simulink model "aaaqi"  (R2016b)
settings: Solver=ode4  StartTime=0.0  StopTime=inf  FixedStep=0.002  RelTol=1e-3  EnableMultiTasking=on
undefined symbols (not defined in the file or in its folder): bit, mdaadlink6208, sigbuilder_block, Standard
libraries: slrtlib x20, slrtsoftinglib x11, simulink x10
(part 4 of 4)

== stateflow chart aaaqi/Subsystem2/shoudong/Chart ==
  state shoudong
    state kaiguangai [parallel]
      settings: executionOrder=1
      state start
        entry:
        xuansong=0;
        xuanjin=0;
        suoding=0;
        jiesuo=0;
        kaigaikaishi=0;
        guangaikaishi=0;
        diancifa20=0;
      state on1
        entry:diancifa20=1;
      state on5
        entry:
        jiesuo=1;
      state on2
        entry:
        xuansong=1;
      state off10
        entry:
        jiesuo=0;
      state off8
        entry:
        xuansong=0;
      state off5
        entry:
        jiesuo=0;
      state off1
        entry:
        xuansong=0;
      state on6
        entry:
        guangaikaishi=1;
      state off2
        entry:
        diancifa20=0;
        SQshiyabuchangwancheng=1;
      state on73
        entry:
        guangaikaishi=0;
      state on7
        entry:
        guangaikaishi=0;
      state on3
        entry:
        kaigaikaishi=1;
      state on71
        entry:
        diancifa20=1;
      state on72
        entry:
        kaigaikaishi=0;
      state on8
        entry:
        xuanjin=1;
      state on4
        entry:
        kaigaikaishi=0;
      state off11
        entry:
        xuanjin=0;
      state on41
        entry:
        suoding=1;
      state off6
        entry:
        xuanjin=0;
      state off9
        entry:
        suoding=0;
      state off3
        entry:
        suoding=0;
      state off7
        entry:
        diancifa20=0;
        SQxuanjinjianyawancheng=1;
        guangaiwancheng=1;
      state off4
        entry:
        kaigaiwancheng=1;
      (default) -> shoudong.kaiguangai.start
      off7 -> shoudong.kaiguangai.start
      shoudong.kaiguangai.start -> shoudong.kaiguangai.on1 : [shiyabuchang==1]
      shoudong.kaiguangai.off4 -> shoudong.kaiguangai.on5 : [jiesuomingling==1]
      off10 -> shoudong.kaiguangai.on5 : [jiesuomingling==1]
      shoudong.kaiguangai.on5 -> (junction 1244)
      shoudong.kaiguangai.on1 -> shoudong.kaiguangai.on2 : [liuliangji==1&&p1>=p2-0.01&&p1<=p2+0.01&&xuansongmingling==1]
      off8 -> shoudong.kaiguangai.on2 : [xuansongmingling==1]
      (junction 1244) -> off10 [order 2] : [jiesuomingling==0]
      (junction 1244) -> off5 [order 1] : [jiesuodaowei1==1&&jiesuodaowei2==1]
      shoudong.kaiguangai.on2 -> (junction 1245)
      (junction 1245) -> off8 [order 2] : [xuansongmingling==0]
      (junction 1245) -> shoudong.kaiguangai.off1 [order 1] : [xuansongdaowei1==1&&xuansongdaowei2==1]
      off5 -> shoudong.kaiguangai.on6 : after(500,tick)[guangai==1]
      shoudong.kaiguangai.off1 -> shoudong.kaiguangai.off2 : after(200,tick)
      on73 -> shoudong.kaiguangai.on6 : [guangai==1]
      shoudong.kaiguangai.on6 -> (junction 1246)
      (junction 1246) -> on73 [order 2] : [guangai==0]
      (junction 1246) -> on7 [order 1] : [guangaijieshu==1]
      shoudong.kaiguangai.off2 -> shoudong.kaiguangai.on3 : after(500,tick)[kaigai==1]
      on7 -> on71 : [xuanjinjianya==1]
      on72 -> shoudong.kaiguangai.on3 : [kaigai==1]
      shoudong.kaiguangai.on3 -> (junction 1247)
      on71 -> on8 : [xuanjinmingling==1]
      (junction 1247) -> on72 [order 2] : [kaigai==0]
      (junction 1247) -> shoudong.kaiguangai.on4 [order 1] : [kaigaijieshu==1]
      off11 -> on8 : [xuanjinmingling==1]
      on8 -> (junction 1248)
      shoudong.kaiguangai.on4 -> on41 : [suodingmingling==1]
      (junction 1248) -> off11 [order 2] : [xuanjinmingling==0]
      (junction 1248) -> shoudong.kaiguangai.off6 [order 1] : [xuanjindaowei1==1&&xuanjindaowei2==1]
      off9 -> on41 : [suoding==1]
      on41 -> (junction 1249)
      (junction 1249) -> off9 [order 2] : [suoding==0]
      (junction 1249) -> shoudong.kaiguangai.off3 [order 1] : [suodingdaowei1==1&&suodingdaowei2==1]
      shoudong.kaiguangai.off6 -> off7 : after(200,tick)
      shoudong.kaiguangai.off3 -> shoudong.kaiguangai.off4 : after(200,tick)
    state SXQxieya [parallel]
      settings: executionOrder=4
      state off1
        entry:
        diancifa11_1=0;
        diancifa11_5=0;
        bililiuliangfa18_1=0;
        bililiuliangfa18_2=0;
        bililiuliangfa18_3=0;
        bililiuliangfa18_4=0;
      state on1
        entry:
        diancifa11_5=1;
      state xieya1
        entry:
        bililiuliangfa18_1=1;
        bililiuliangfa18_2=1;
        p0_2=p0sheding;
      state xieya1_1
        entry:
        bililiuliangfa18_1=1;
        bililiuliangfa18_2=1;
      state xieya1_2
        entry:
        bililiuliangfa18_1=1;
        bililiuliangfa18_2=0;
      state xieya2
        entry:
        bililiuliangfa18_1=1;
        bililiuliangfa18_2=1;
        p0_2=p0_2-0.03;
      state xieya1_3
        entry:
        bililiuliangfa18_1=0;
        bililiuliangfa18_2=1;
      state xieya7_1
        entry:
        bililiuliangfa18_1=1;
        bililiuliangfa18_2=1;
      state xieya7_2
        entry:
        bililiuliangfa18_1=1;
        bililiuliangfa18_2=0;
      state xieya8
        entry:
        bililiuliangfa18_1=1;
        bililiuliangfa18_2=1;
      state xieya7_3
        entry:
        bililiuliangfa18_1=0;
        bililiuliangfa18_2=1;
      state off2
        entry:
        diancifa11_5=0;
        bililiuliangfa18_1=0;
        bililiuliangfa18_2=0;
        SXQxieyawancheng=1;
      (default) -> shoudong.SXQxieya.off1
      (junction 1418) -> shoudong.SXQxieya.off1
      (junction 1419) -> shoudong.SXQxieya.off1
      (junction 1421) -> (junction 1418) [order 2] : [SXQxieya==0]
      (junction 1424) -> (junction 1418) [order 2] : [SXQxieya==0]
      (junction 1420) -> (junction 1418) [order 2] : [SXQxieya==0]
      (junction 1423) -> (junction 1418) [order 2] : [SXQxieya==0]
      (junction 1426) -> (junction 1419) [order 2] : [SXQxieya==0]
      (junction 1429) -> (junction 1419) [order 2] : [SXQxieya==0]
      (junction 1427) -> (junction 1419) [order 2] : [SXQxieya==0]
      (junction 1430) -> (junction 1419) [order 2] : [SXQxieya==0]
      shoudong.SXQxieya.off1 -> shoudong.SXQxieya.on1 : [SXQxieya==1]
      shoudong.SXQxieya.on1 -> xieya1 : after(500,tick)
      xieya1 -> (junction 1422)
      (junction 1422) -> (junction 1421) [order 2] : [p2<=p0_2&&p3>p0_2]
      (junction 1420) -> xieya1_1 [order 1] : [SXQxieya==1]
      (junction 1421) -> xieya1_2 [order 1] : [SXQxieya==1]
      (junction 1422) -> (junction 1420) [order 1] : [p2>p0_2&&p3>p0_2]
      xieya1_2 -> (junction 1422)
      xieya1_1 -> (junction 1422)
      xieya1_3 -> (junction 1422)
      (junction 1422) -> (junction 1423) [order 4] : [p2<=p0_2&&p3<=p0_2]
      (junction 1422) -> (junction 1424) [order 3] : [p2>p0_2&&p3<=p0_2]
      (junction 1425) -> (junction 1422) [order 2] : [p0_2>p0_0]
      (junction 1423) -> xieya2 [order 1] : [SXQxieya==1]
      (junction 1424) -> xieya1_3 [order 1] : [SXQxieya==1]
      xieya2 -> (junction 1425)
      (junction 1425) -> (junction 1428) [order 1] : [p0_2<=p0_0]
      (junction 1427) -> xieya7_2 [order 1] : [SXQxieya==1]
      (junction 1426) -> xieya7_1 [order 1] : [SXQxieya==1]
      (junction 1428) -> (junction 1427) [order 2] : [p2<=p0_0&&p3>p0_0]
      (junction 1428) -> (junction 1426) [order 1] : [p2>p0_0&&p3>p0_0]
      xieya7_1 -> (junction 1428)
      xieya7_2 -> (junction 1428)
      (junction 1428) -> (junction 1430) [order 3] : [p2>p0_0&&p3<=p0_0]
      (junction 1428) -> (junction 1429) [order 4] : [p2<=p0_0&&p3<=p0_0]
      xieya7_3 -> (junction 1428)
      (junction 1431) -> (junction 1428) [order 2] : [p2>p0_0||p3>p0_0]
      (junction 1429) -> xieya8 [order 1] : [SXQxieya==1]
      (junction 1430) -> xieya7_3 [order 1] : [SXQxieya==1]
      xieya8 -> (junction 1431) : after(1000,tick)
      (junction 1431) -> shoudong.SXQxieya.off2 [order 1] : [p2<=p0_0&&p3<=p0_0]
    state SCjiaya [parallel]
      settings: executionOrder=2
      state off1
        entry:diancifa11_1=0;
        diancifa11_2=0;
        diancifa16_1=0;
      state on1
        entry:diancifa11_1=1;
        diancifa11_2=1;
        diancifa16_1=0;
      state off2
        entry:
        diancifa11_1=0;
        diancifa11_2=0;
        diancifa16_1=0;
      state on3
        entry:diancifa11_1=1;
        diancifa11_2=1;
        diancifa16_1=0;
      state on2
        entry:diancifa16_1=1;
      state off3
        entry:
        diancifa11_1=0;
        diancifa11_2=0;
        diancifa16_1=0;
      state off4
        entry:
        SCjiayawancheng=1;
      (default) -> shoudong.SCjiaya.off1
      (junction 1311) -> shoudong.SCjiaya.off1
      shoudong.SCjiaya.off1 -> shoudong.SCjiaya.on1 : [SCjiaya==1]
      shoudong.SCjiaya.on1 -> (junction 1312)
      (junction 1312) -> (junction 1311) [order 2] : [SCjiaya==0]
      (junction 1313) -> (junction 1311) [order 2] : [SCjiaya==0]
      (junction 1312) -> shoudong.SCjiaya.off2 [order 1] : [p1>=p1sheding]
      shoudong.SCjiaya.off2 -> (junction 1313)
      shoudong.SCjiaya.on3 -> (junction 1314)
      (junction 1313) -> (junction 1314) [order 1] : after(1000,tick)
      shoudong.SCjiaya.on2 -> (junction 1314)
      (junction 1314) -> shoudong.SCjiaya.on2 [order 2] : [p1>p1sheding+0.005]
      (junction 1314) -> shoudong.SCjiaya.on3 [order 1] : [p1<p1sheding]
      (junction 1314) -> shoudong.SCjiaya.off3 [order 3] : [p1>=p1sheding&&p1<=p1sheding+0.005]
      shoudong.SCjiaya.off3 -> shoudong.SCjiaya.off4
    state SCzhushui [parallel]
      settings: executionOrder=3
      state off4
        entry:diancifa16_1=0;
        diancifa3=0;
      state on2
        entry:diancifa16_1=1;
      state on3
        entry:diancifa3=1;
      state off1
        entry:diancifa3=0;
      state off2
        entry:diancifa16_1=0;
      state off3
        entry:
        SCzhushuiwancheng=1;
      (default) -> shoudong.SCzhushui.off4
      (junction 1338) -> shoudong.SCzhushui.off4 [order 2] : [SCzhushui==0]
      shoudong.SCzhushui.off4 -> shoudong.SCzhushui.on2 : [SCzhushui==1]
      shoudong.SCzhushui.on2 -> shoudong.SCzhushui.on3 : after(20,tick)
      shoudong.SCzhushui.on3 -> (junction 1338)
      (junction 1338) -> shoudong.SCzhushui.off1 [order 1] : [fuqiuyeweikongzhiqi==1]
      shoudong.SCzhushui.off1 -> shoudong.SCzhushui.off2
      shoudong.SCzhushui.off2 -> shoudong.SCzhushui.off3
    state SXQjunya [parallel]
      settings: executionOrder=5
      state jiaya1_1
        entry:
        bililiuliangfa18_3=1;
        bililiuliangfa18_4=1;
      state jiaya7_1
        entry:
        bililiuliangfa18_3=1;
        bililiuliangfa18_4=1;
      state jiaya7_3
        entry:
        bililiuliangfa18_3=0;
        bililiuliangfa18_4=1;
      state on6
        entry:
        bililiuliangfa18_3=1;
        diancifa3=1;
        p0_1=p0_1+0.02;
      state on5
        entry:
        bililiuliangfa18_3=1;
        diancifa3=1;
      state jiaya2
        entry:
        bililiuliangfa18_3=1;
        bililiuliangfa18_4=1;
        p0_1=p0_1+0.03;
      state off1
        entry:
        diancifa11_1=0;
        diancifa11_5=0;
        diancifa20=0;
        diancifa3=0;
        bililiuliangfa18_1=0;
        bililiuliangfa18_2=0;
        bililiuliangfa18_3=0;
        bililiuliangfa18_4=0;
      state jiaya1
        entry:
        diancifa3=0;
        bililiuliangfa18_3=1;
        bililiuliangfa18_4=1;
        p0_1=p0sheding_qi;
      state on1
        entry:
        diancifa11_1=1;
      state on2
        entry:
        bililiuliangfa18_3=1;
        diancifa3=1;
      state jiaya7_2
        entry:
        bililiuliangfa18_3=1;
        bililiuliangfa18_4=0;
      state jiaya1_2
        entry:
        bililiuliangfa18_3=1;
        bililiuliangfa18_4=0;
      state on3
        entry:
        bililiuliangfa18_3=0;
        diancifa3=1;
      state on4
        entry:
        bililiuliangfa18_3=1;
        diancifa3=0;
      state jiaya1_3
        entry:
        bililiuliangfa18_3=0;
        bililiuliangfa18_4=1;
      state off4
        entry:
        bililiuliangfa18_3=0;
        bililiuliangfa18_4=0;
      state off3
        entry:
        bililiuliangfa18_1=0;
        bililiuliangfa18_2=0;
      state off2
        entry:
        bililiuliangfa18_1=0;
        bililiuliangfa18_2=0;
        bililiuliangfa18_3=0;
        bililiuliangfa18_4=0;
      state jiance1_34
        entry:
        bililiuliangfa18_1=1;
        bililiuliangfa18_2=0;
      state jiance1_32
        entry:
        bililiuliangfa18_1=1;
        bililiuliangfa18_2=1;
      state jiance1_36
        entry:
        bililiuliangfa18_1=0;
        bililiuliangfa18_2=1;
      state off6
        entry:
        diancifa11_1=0;
        diancifa11_5=0;
        SXQjunyawancheng=1;
      jiaya1_1 -> (junction 1492)
      (junction 1683) -> shoudong.SXQjunya.on6 [order 1] : [SXQjunya==1]
      jiaya7_3 -> (junction 1494)
      shoudong.SXQjunya.on5 -> (junction 1665)
      (junction 1488) -> jiaya2 [order 1] : [SXQjunya==1]
      (junction 1487) -> jiaya7_1 [order 1] : [SXQjunya==1]
      (default) -> shoudong.SXQjunya.off1
      (junction 1490) -> jiaya1_1 [order 1] : [SXQjunya==1]
      jiaya7_1 -> (junction 1494)
      (junction 1489) -> jiaya7_3 [order 1] : [SXQjunya==1]
      (junction 1684) -> shoudong.SXQjunya.on5 [order 1] : [SXQjunya==1]
      shoudong.SXQjunya.on6 -> (junction 1676)
      (junction 1487) -> (junction 1499) [order 2] : [SXQjunya==0]
      (junction 1494) -> (junction 1487) [order 1] : [p2<p0sheding&&p3<p0sheding]
      jiaya2 -> (junction 1493)
      (junction 1665) -> (junction 1683) [order 4] : [p2>=p0_1&&p3>=p0_1]
      (junction 1683) -> (junction 1666) [order 2] : [SXQjunya==0]
      (junction 1492) -> (junction 1488) [order 4] : [p2>=p0_1&&p3>=p0_1]
      (junction 1488) -> (junction 1498) [order 2] : [SXQjunya==0]
      (junction 1489) -> (junction 1499) [order 2] : [SXQjunya==0]
      (junction 1494) -> (junction 1489) [order 3] : [p2<p0sheding&&p3>=p0sheding]
      (junction 1665) -> (junction 1684) [order 1] : [p2<p0_1&&p3<p0_1]
      (junction 1492) -> (junction 1490) [order 1] : [p2<p0_1&&p3<p0_1]
      (junction 1490) -> (junction 1498) [order 2] : [SXQjunya==0]
      (junction 1684) -> (junction 1666) [order 2] : [SXQjunya==0]
      (junction 1494) -> (junction 1491) [order 2] : [p2>=p0sheding&&p3<p0sheding]
      (junction 1491) -> (junction 1499) [order 2] : [SXQjunya==0]
      (junction 1491) -> jiaya7_2 [order 1] : [SXQjunya==1]
      jiaya1 -> (junction 1492)
      (junction 1493) -> (junction 1492) [order 2] : [p0_1<p0sheding]
      (junction 1493) -> (junction 1494) [order 1] : [p0_1>=p0sheding]
      shoudong.SXQjunya.on1 -> shoudong.SXQjunya.on2 : after(500,tick)
      (junction 1492) -> (junction 1496) [order 3] : [p2<p0_1&&p3>=p0_1]
      jiaya7_2 -> (junction 1494)
      jiaya1_3 -> (junction 1492)
      shoudong.SXQjunya.on2 -> (junction 1665)
      (junction 1676) -> (junction 1665) [order 2] : [p0_1<=p0sheding_qi]
      (junction 1676) -> jiaya1 [order 1] : [p0_1>p0sheding_qi]
      shoudong.SXQjunya.off3 -> (junction 1494) [order 2] : [p2<=(p0sheding+0.005)&&p3<=(p0sheding+0.005)]
      (junction 1492) -> (junction 1495) [order 2] : [p2>=p0_1&&p3<p0_1]
      shoudong.SXQjunya.off1 -> shoudong.SXQjunya.on1 : [SXQjunya==1]
      shoudong.SXQjunya.off4 -> (junction 1494) [order 2] : [p2<p0sheding||p3<p0sheding]
      jiaya1_2 -> (junction 1492)
      (junction 1494) -> (junction 1497) [order 4] : after(250,tick)[p2>=p0sheding&&p3>=p0sheding]
      (junction 1665) -> (junction 1670) [order 2] : [p2<p0_1&&p3>=p0_1]
      (junction 1665) -> (junction 1680) [order 3] : [p2>=p0_1&&p3<p0_1]
      shoudong.SXQjunya.on4 -> (junction 1665)
      shoudong.SXQjunya.on3 -> (junction 1665)
      (junction 1495) -> jiaya1_2 [order 1] : [SXQjunya==1]
      (junction 1495) -> (junction 1498) [order 2] : [SXQjunya==0]
      (junction 1496) -> jiaya1_3 [order 1] : [SXQjunya==1]
      (junction 1680) -> shoudong.SXQjunya.on4 [order 1] : [SXQjunya==1]
      (junction 1496) -> (junction 1498) [order 2] : [SXQjunya==0]
      (junction 1680) -> (junction 1666) [order 2] : [SXQjunya==0]
      (junction 1670) -> shoudong.SXQjunya.on3 [order 1] : [SXQjunya==1]
      (junction 1670) -> (junction 1666) [order 2] : [SXQjunya==0]
      (junction 1666) -> shoudong.SXQjunya.off1
      (junction 1497) -> (junction 1499) [order 2] : [SXQjunya==0]
      (junction 1497) -> shoudong.SXQjunya.off4 [order 1] : [SXQjunya==1]
      (junction 1500) -> shoudong.SXQjunya.off3 [order 1] : [SXQjunya==1]
      (junction 1499) -> (junction 1498)
      (junction 1498) -> (junction 1666)
      (junction 1501) -> (junction 1499)
      shoudong.SXQjunya.off3 -> (junction 1503) [order 1] : [p2>(p0sheding+0.005)||p3>(p0sheding+0.005)]
      shoudong.SXQjunya.off4 -> (junction 1503) [order 1]
      (junction 1500) -> (junction 1501) [order 2] : [SXQjunya==0]
      (junction 1503) -> (junction 1500) [order 5] : after(250,tick)[p2<=(p0sheding+0.005)&&p3<=(p0sheding+0.005)]
      (junction 1502) -> (junction 1501) [order 2] : [SXQjunya==0]
      (junction 1504) -> (junction 1501) [order 2] : [SXQjunya==0]
      (junction 1506) -> (junction 1501) [order 2] : [SXQjunya==0]
      (junction 1503) -> (junction 1502) [order 1] : [p2<=(p0sheding+0.005)&&p3>(p0sheding+0.005)]
      (junction 1502) -> jiance1_34 [order 1] : [SXQjunya==1]
      (junction 1503) -> shoudong.SXQjunya.off2 [order 2] : [p2>=p0sheding&&p3>=p0sheding&&p2<=(p0sheding+0.005)&&p3<=(p0sheding+0.005)]
      jiance1_34 -> (junction 1503)
      (junction 1505) -> (junction 1503) [order 1] : [p2<p0sheding||p2>(p0sheding+0.005)||p3<p0sheding||p3>(p0sheding+0.005)]
      jiance1_32 -> (junction 1503)
      (junction 1503) -> (junction 1504) [order 3] : [p2>(p0sheding+0.005)&&p3<=(p0sheding+0.005)]
      jiance1_36 -> (junction 1503)
      (junction 1503) -> (junction 1506) [order 4] : [p2>(p0sheding+0.005)&&p3>(p0sheding+0.005)]
      shoudong.SXQjunya.off2 -> (junction 1505) : after(1000,tick)
      (junction 1504) -> jiance1_36 [order 1] : [SXQjunya==1]
      (junction 1505) -> shoudong.SXQjunya.off6 [order 2] : [p2>=p0sheding&&p2<=(p0sheding+0.005)&&p3>=p0sheding&&p3<=(p0sheding+0.005)]
      (junction 1506) -> jiance1_32 [order 1] : [SXQjunya==1]
  state start
    en:
    diancifa11_1=0;
    diancifa11_2=0;
    diancifa11_5=0;
    diancifa20=0;
    diancifa16_1=0;
    diancifa3=0;
    diancifa21=0;
    bililiuliangfa18_1=0;
    bililiuliangfa18_2=0;
    bililiuliangfa18_3=0;
    bililiuliangfa18_4=0;
    xuansong=0;
    xuanjin=0;
    suoding=0;
    jiesuo=0;
    kaigaikaishi=0;
    guangaikaishi=0;
  state off111
    en:
    diancifa11_1=0;
    diancifa11_2=0;
    diancifa11_5=0;
    diancifa20=0
    diancifa16_1=0;
    diancifa3=0;
    diancifa21=0;
    bililiuliangfa18_1=0;
    bililiuliangfa18_2=0;
    bililiuliangfa18_3=0;
    bililiuliangfa18_4=0;
    xuansong=0;
    xuanjin=0;
    suoding=0;
    jiesuo=0;
    SCzhushuiwancheng=0;
    SCjiayawancheng=0;
    SXQjunyawancheng=0;
    SQshiyabuchangwancheng=0;
    kaigaikaishi=0;
    kaigaiwancheng=0;
    SQxuanjinjianyawancheng=0;
    guangaikaishi=0;
    guangaiwancheng=0;
    SXQxieyawancheng=0;
  (default) -> start
  start -> shoudong : [start==1]
  off111 -> start : [start==0&&jiting==0]
  shoudong -> off111 : [jiting==1||start==0]
  data: start input double; diancifa11_1 output double; diancifa11_2 output double; diancifa11_5 output double; SCzhushui input double; fuqiuyeweikongzhiqi input double; diancifa20 output double; diancifa16_1 output double; diancifa3 output double; SCjiaya input double; SXQjunya input double; diancifa21 output double; suoding output double; jiesuo output double; xuansong output double; xuanjin output double; bililiuliangfa18_1 output double; bililiuliangfa18_2 output double; bililiuliangfa18_3 output double; bililiuliangfa18_4 output double; SXQxieya input double; p1 input double; p1sheding input double; liuliangji input double; p2 input double; p3 input double; p0_0 input double; p0sheding input double; kaigaikaishi output double; guangaikaishi output double; SCzhushuiwancheng output double; SCjiayawancheng output double; SXQjunyawancheng output double; SXQxieyawancheng output double; SQshiyabuchangwancheng output double; SQxuanjinjianyawancheng output double; kaigaiwancheng output double; guangaiwancheng output double; xuansongdaowei1 input double; xuansongdaowei2 input double; xuanjindaowei1 input double; xuanjindaowei2 input double; suodingdaowei1 input double; suodingdaowei2 input double; jiesuodaowei1 input double; jiesuodaowei2 input double; kaigaijieshu input double; guangaijieshu input double; jiting input double; kaigai input double; guangai input double; shiyabuchang input double; xuansongmingling input double; suodingmingling input double; jiesuomingling input double; xuanjinjianya input double; xuanjinmingling input double; p0_1 output double; p0_2 output double; p0sheding_qi input double

== stateflow chart aaaqi/guangaiquxian/Chart1 ==
  state on1
    en:
    x=0;
    t=0;
  state on2
    entry:
    x++;
    t=x*0.002
  (default) -> on1
  (junction 14) -> on1 [order 2] : [a==0]
  on1 -> on2 : [a==1]
  on2 -> (junction 14)
  (junction 14) -> on2 [order 1] : [a==1]
  data: a input double; x local double; t output double

== stateflow chart aaaqi/kaigaiquxian/Chart ==
  state on1
    en:
    x=0;
    t=0;
  state on2
    entry:
    x++;
    t=x*0.002
  (default) -> on1
  (junction 14) -> on1 [order 2] : [a==0]
  on1 -> on2 : [a==1]
  on2 -> (junction 14)
  (junction 14) -> on2 [order 1] : [a==1]
  data: a input double; x local double; t output double
